simulink model "Lab4"  (Simulink 8.4)
settings: Solver=ode45  SolverMode=SingleTasking  StartTime=0.0  StopTime=10.0  RelTol=1e-3  AbsTol=1e-6
settings Model: Creator=vise  LastModifiedBy=M. Cenk Cavusoglu  ExtModeTrigMode=oneshot  ExtModeArmWhenConnect=off
settings DataIOCC: LimitDataPoints=off
settings OptimizationCC: BlockReduction=off  BooleanDataType=off  InitFltsAndDblsToZero=on
settings DebuggingCC: SaveWithParameterizedLinksMsg=none  SignalResolutionControl=TryResolveAllWithWarning  SolverPrmCheckMsg=none  MultiTaskDSMMsg=warning  MultiTaskCondExecSysMsg=none  StrictBusMsg=None
settings HardwareCC: TargetUnknown=on
settings RTWCC: TemplateMakefile=grt_unix.tmf  IncludeERTFirstTime=on

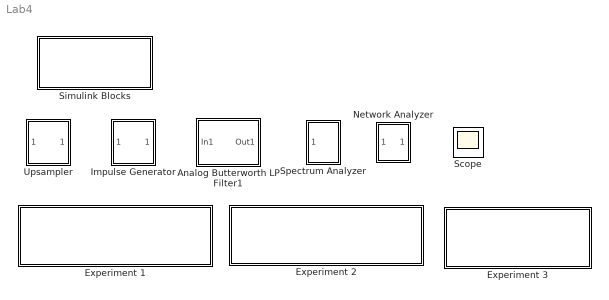
== system Lab4 ==
  Analog Butterworth LP Filter1 : Subsystem  mask(buttap){MaskParam1=2*pi, MaskParam2=10}
      mask prompts: MaskParam1 "Cutoff frequency (rad/sec)"; MaskParam2 "Order"
      mask help:
      | Analog Butterworth low pass filter.
      |
      | (Requires Signal Processing Toolbox)
      mask init:
      | [z,p,k]=buttap(MaskParam2); z=MaskParam1*z; p=MaskParam1*p; k=real(prod(-p)); [num,den]=zp2tf(z,p,k); w=logspace(log10(MaskParam1/10),log10(10*MaskParam1),20); h=freqs(num,den,w);
      mask Help: Butterworth low pass filter using MATLAB's butter command.
      mask Display: plot(20*log10(w),20*log10(abs(h)))
  Experiment 1 : Subsystem  mask(Impulse Generator){}
      settings: OpenFcn=ImpulseGen
      mask Display: disp('Sampling and Reconstruction \n Using an Inpulse Generator')
  Experiment 2 : Subsystem  mask(Sample and Hold){}
      settings: OpenFcn=SampHold
      mask Display: disp('Sampling and Reconstruction \nUsing a Sample and Hold')
  Experiment 3 : Subsystem  mask(Interpolator){}
      settings: OpenFcn=Interp
      mask Display: disp('Discrete Time \nInterpolator')
  Impulse Generator : Subsystem  mask(D-T interpolator){T=1, MaskParam2=0.2}
      mask prompts: T "Input sampling period:"; MaskParam2 "Pulse width:"
      mask init:
      | L=round(T/MaskParam2);
      mask Display: plot(-10,-10,110,110,[0,50,50,60,60,100],[0,0,80,80,0,0])
  Network Analyzer : Subsystem  mask(Network Analyzer){MaskParam1=256, MaskParam2=0.1}
      mask prompts: MaskParam1 "Number of sample points:"; MaskParam2 "Sampling period (sec):"
      mask init:
      | max_freq=0.9*pi/MaskParam2;N=MaskParam1;T_s=MaskParam2;const=2*pi/(MaskParam1*MaskParam2);window1=0.5*MaskParam1*MaskParam2;window2=MaskParam1*MaskParam2;
      mask Help: Estimates frequency response of system using chirp input. Used for EE438. See Prof. Bouman.
      mask Display: plot(0,0,100,100,[11,93,93,11,11],[90,90,40,40,90],[80,60,40,20],[50,79,50,80])
  Scope : Scope
      settings: TickLabels=on
  Simulink Blocks : Subsystem  mask(Waveform Synthesizer){}
      settings: OpenFcn=simulink
      mask Display: disp('Full Block Library')
  Spectrum Analyzer : Subsystem  mask(Spectrum analyzer.){N=2048, T_s=0.02, plot_period=10}
      mask prompts: N "Number of sample points:"; T_s "Sampling period (sec):"; plot_period "Plotting Period (sec):"
      mask Help: EE438 Lab utility; See Prof. Bouman.
      mask Display: plot(0,0,100,100,[14,91,91,14,14],[86,86,40,40,86],[85,82,80,79,75,67,63,60,57,53,41,36,33,27,24],[49,50,53,50,49,51,54,66,54,50,50,52,81,51,49])
  Upsampler : Subsystem  mask(D-T interpolator){T=1, L=1}
      mask prompts: T "Input sampling period:"; L "Upsampling factor:"
      mask Display: disp('L')

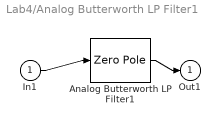
== system Lab4/Analog Butterworth LP Filter1 ==
  In1 : Inport
  Analog Butterworth LP Filter1 : ZeroPole  Zeros=z  Poles=p  Gain=k
  Out1 : Outport
  wires:
  In1/1 -> Analog Butterworth LP Filter1/1
  Analog Butterworth LP Filter1/1 -> Out1/1

== system Lab4/Experiment 1 ==

== system Lab4/Experiment 2 ==

== system Lab4/Experiment 3 ==

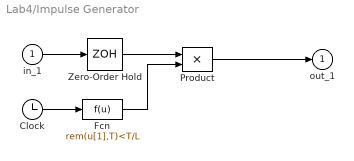
== system Lab4/Impulse Generator ==
  in_1 : Inport
  Clock : Clock
  Fcn : Fcn  Expr=rem(u[1],T)<T/L
  Product : Product  SaturateOnIntegerOverflow=on  RndMeth=Zero  InputSameDT=on  OutDataTypeStr=Inherit: Same as first input
  Zero-Order Hold : ZeroOrderHold  SampleTime=T
  out_1 : Outport  InitialOutput=0
  wires:
  in_1/1 -> Zero-Order Hold/1
  Zero-Order Hold/1 -> Product/1
  Fcn/1 -> Product/2
  Product/1 -> out_1/1
  Clock/1 -> Fcn/1

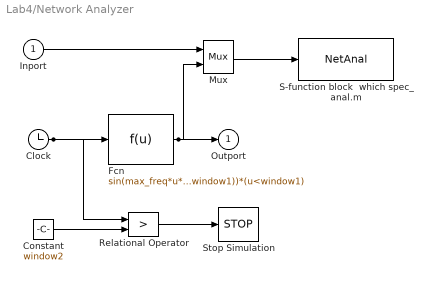
== system Lab4/Network Analyzer ==
  Inport : Inport
  Clock : Clock
  Constant : Constant  Value=window2
  Fcn : Fcn  Expr=sin(max_freq*u*u/(2*window1))*(0.54+0.46*cos(pi*u/window1))*(u<window1)
  Mux : Mux  Inputs=2
  Relational Operator : RelationalOperator  Operator=>  InputSameDT=on
  S-function block  which spec_anal.m : S-Function  FunctionName=NetAnal  Parameters=N,T_s  EnableBusSupport=off
  Stop Simulation : Stop
  Outport : Outport  InitialOutput=0
  wires:
  Inport/1 -> Mux/1
  Fcn/1 -> Mux/2, Outport/1
  Mux/1 -> S-function block  which spec_anal.m/1
  Clock/1 -> Fcn/1, Relational Operator/1
  Constant/1 -> Relational Operator/2
  Relational Operator/1 -> Stop Simulation/1

== system Lab4/Simulink Blocks ==

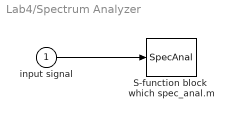
== system Lab4/Spectrum Analyzer ==
  input signal : Inport
  S-function block  which spec_anal.m : S-Function  FunctionName=SpecAnal  Parameters=N,T_s,plot_period  EnableBusSupport=off
  wires:
  input signal/1 -> S-function block  which spec_anal.m/1

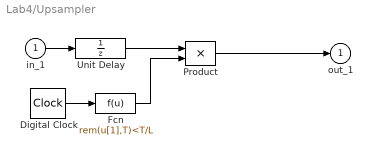
== system Lab4/Upsampler ==
  in_1 : Inport
  Digital Clock : DigitalClock  SampleTime=T/L
  Fcn : Fcn  Expr=rem(u[1],T)<T/L
  Product : Product  SaturateOnIntegerOverflow=on  RndMeth=Zero  InputSameDT=on  OutDataTypeStr=Inherit: Same as first input
  Unit Delay : UnitDelay  SampleTime=T/L
  out_1 : Outport  InitialOutput=0
  wires:
  Product/1 -> out_1/1
  Fcn/1 -> Product/2
  Unit Delay/1 -> Product/1
  in_1/1 -> Unit Delay/1
  Digital Clock/1 -> Fcn/1
